simulink model "test"  (R2023a)
settings: Solver=FixedStepAuto  StartTime=0.0  StopTime=1  FixedStep=1e-4  MaxStep=1e-4  MinStep=1e-5  RelTol=1e-6  AbsTol=1e-5
values from neighbouring files (symbols this model uses):
  abc_alpha_beta = sqrt(2/3) * [1, -1/2, -1/2 ... (first row only)    [main.m]
  Flux_1 = 1/(Msr^2 - Ls * Lr )  * [Rs*Lr, 0, -Rs*Msr, 0 ... (first row only)    [main.m]
  Flux_2 = 1/(Msr^2 - Ls * Lr )  * [0, 0, 0, 0 ... (first row only)    [main.m]
  frot = 0.01    [main.m]
  Inv_abc_alpha_beta = inv(abc_alpha_beta)    [main.m]
  Inv_Phi_Courant = inv(Phi_Courant)    [main.m]
  J = 0.025    [main.m]
  Lr = 0.194    [main.m]
  Ls = 0.182    [main.m]
  Msr = 0.182    [main.m]
  p = 2    [main.m]
  Rr = 1.15    [main.m]
  Rs = 1.6    [main.m]
  T_charge = 0    [main.m]
  Vn = 380    [main.m]
settings Model: Creator=philippecasteres  LastModifiedBy=philippecasteres

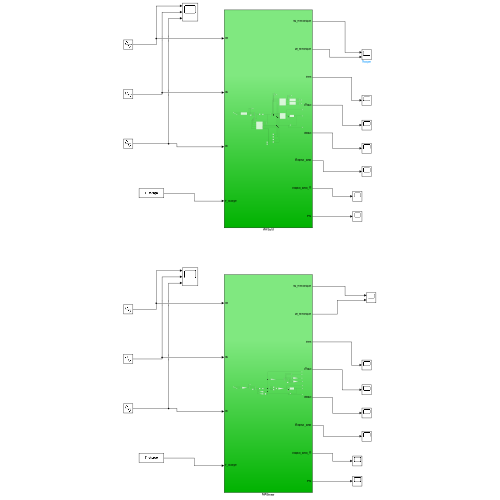
[thumbnail: Simulink's stored preview of the top-level diagram]
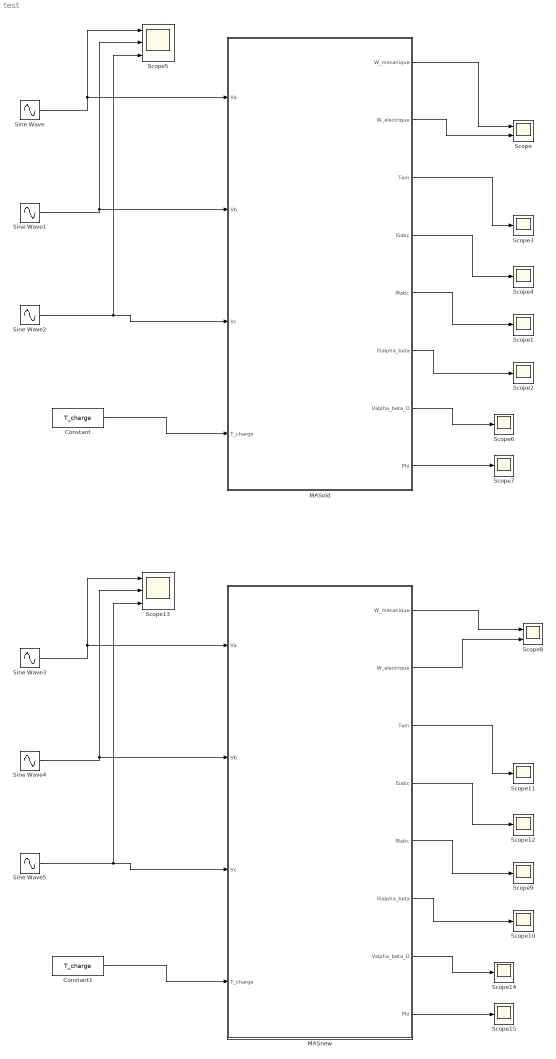
== system test ==
  Constant : Constant  Value=T_charge
  Constant1 : Constant  Value=T_charge
  MASnew : Subsystem
  MASold : Subsystem
  Scope : Scope  NumInputPorts=2
  Scope{1..4,6..7,9..12,14..15} (12 alike) : Scope
  Scope13 : Scope  NumInputPorts=3
  Scope5 : Scope  NumInputPorts=3
  Scope8 : Scope  NumInputPorts=2
  Sine Wave : Sin  Amplitude=Vn  Frequency=50*2*pi  SampleTime=0
  Sine Wave1 : Sin  Amplitude=Vn  Frequency=50*2*pi  Phase=-2*pi/3  SampleTime=0
  Sine Wave2 : Sin  Amplitude=Vn  Frequency=50*2*pi  Phase=-4*pi/3  SampleTime=0
  Sine Wave3 : Sin  Amplitude=Vn  Frequency=50*2*pi  SampleTime=0
  Sine Wave4 : Sin  Amplitude=Vn  Frequency=50*2*pi  Phase=-2*pi/3  SampleTime=0
  Sine Wave5 : Sin  Amplitude=Vn  Frequency=50*2*pi  Phase=-4*pi/3  SampleTime=0
  wires:
  Sine Wave2/1 -> Scope5/3, MASold/3(Vc)
  Sine Wave1/1 -> Scope5/2, MASold/2(Vb)
  Sine Wave/1 -> Scope5/1, MASold/1(Va)
  MASold/1(W_mecanique) -> Scope/1
  MASold/2(W_electrique) -> Scope/2
  MASold/3(Tem) -> Scope3/1
  Constant/1 -> MASold/4(T_charge)
  MASold/4(ISabc) -> Scope4/1
  MASold/5(IRabc) -> Scope1/1
  MASold/6(ISalpha_beta) -> Scope2/1
  MASold/7(Valpha_beta_O) -> Scope6/1
  MASold/8(Phi) -> Scope7/1
  MASnew/2(W_electrique) -> Scope8/2
  Sine Wave3/1 -> MASnew/1(Va), Scope13/1
  MASnew/1(W_mecanique) -> Scope8/1
  Sine Wave4/1 -> MASnew/2(Vb), Scope13/2
  MASnew/3(Tem) -> Scope11/1
  Constant1/1 -> MASnew/4(T_charge)
  Sine Wave5/1 -> MASnew/3(Vc), Scope13/3
  MASnew/4(ISabc) -> Scope12/1
  MASnew/7(Valpha_beta_O) -> Scope14/1
  MASnew/5(IRabc) -> Scope9/1
  MASnew/6(ISalpha_beta) -> Scope10/1
  MASnew/8(Phi) -> Scope15/1

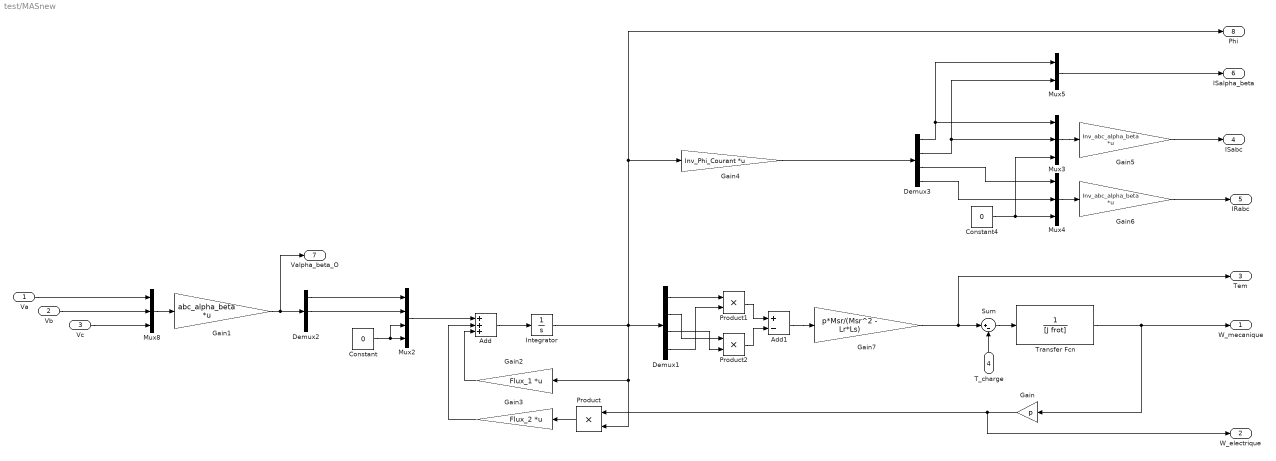
== system test/MASnew ==
  Va : Inport
  Vb : Inport  Port=2
  Vc : Inport  Port=3
  T_charge : Inport  Port=4
  Add : Sum  Inputs=+++
  Add1 : Sum  Inputs=+-
  Constant : Constant  Value=0
  Constant4 : Constant  Value=0
  Demux1 : Demux
  Demux2 : Demux  Outputs=3
  Demux3 : Demux
  Gain : Gain  Gain=p
  Gain1 : Gain  Gain=abc_alpha_beta  Multiplication=Matrix(K*u)
  Gain2 : Gain  Gain=Flux_1  Multiplication=Matrix(K*u)
  Gain3 : Gain  Gain=Flux_2  Multiplication=Matrix(K*u)
  Gain4 : Gain  Gain=Inv_Phi_Courant  Multiplication=Matrix(K*u)
  Gain5 : Gain  Gain=Inv_abc_alpha_beta  Multiplication=Matrix(K*u)
  Gain6 : Gain  Gain=Inv_abc_alpha_beta  Multiplication=Matrix(K*u)
  Gain7 : Gain  Gain=p*Msr/(Msr^2 - Lr*Ls)
  Integrator : Integrator
  Mux2 : Mux
  Mux3 : Mux  Inputs=3
  Mux4 : Mux  Inputs=3
  Mux5 : Mux  Inputs=2
  Mux8 : Mux  Inputs=3
  Product : Product
  Product1 : Product
  Product2 : Product
  Sum : Sum  Inputs=|+-
  Transfer Fcn : TransferFcn  Denominator=[J frot]
  W_mecanique : Outport
  W_electrique : Outport  Port=2
  Tem : Outport  Port=3
  ISabc : Outport  Port=4
  IRabc : Outport  Port=5
  ISalpha_beta : Outport  Port=6
  Valpha_beta_O : Outport  Port=7
  Phi : Outport  Port=8
  wires:
  Demux3/4 -> Mux4/2
  Demux3/2 -> Mux3/2, Mux5/2
  T_charge/1 -> Sum/2
  Demux3/1 -> Mux3/1, Mux5/1
  Va/1 -> Mux8/1
  Sum/1 -> Transfer Fcn/1
  Demux1/1 -> Product1/1
  Demux3/3 -> Mux4/1
  Gain7/1 -> Sum/1, Tem/1
  Transfer Fcn/1 -> Gain/1, W_mecanique/1
  Add/1 -> Integrator/1
  Vc/1 -> Mux8/3
  Vb/1 -> Mux8/2
  Product/1 -> Gain3/1
  Integrator/1 -> Gain2/1, Product/2, Demux1/1, Gain4/1, Phi/1
  Mux2/1 -> Add/1
  Mux3/1 -> Gain5/1
  Mux5/1 -> ISalpha_beta/1
  Gain1/1 -> Valpha_beta_O/1, Demux2/1
  Mux8/1 -> Gain1/1
  Demux2/1 -> Mux2/1
  Demux2/2 -> Mux2/2
  Constant/1 -> Mux2/4, Mux2/3
  Gain2/1 -> Add/3
  Gain4/1 -> Demux3/1
  Constant4/1 -> Mux4/3, Mux3/3
  Gain5/1 -> ISabc/1
  Mux4/1 -> Gain6/1
  Gain6/1 -> IRabc/1
  Product1/1 -> Add1/1
  Product2/1 -> Add1/2
  Add1/1 -> Gain7/1
  Gain/1 -> W_electrique/1, Product/1
  Gain3/1 -> Add/2
  Demux1/4 -> Product1/2
  Demux1/2 -> Product2/1
  Demux1/3 -> Product2/2

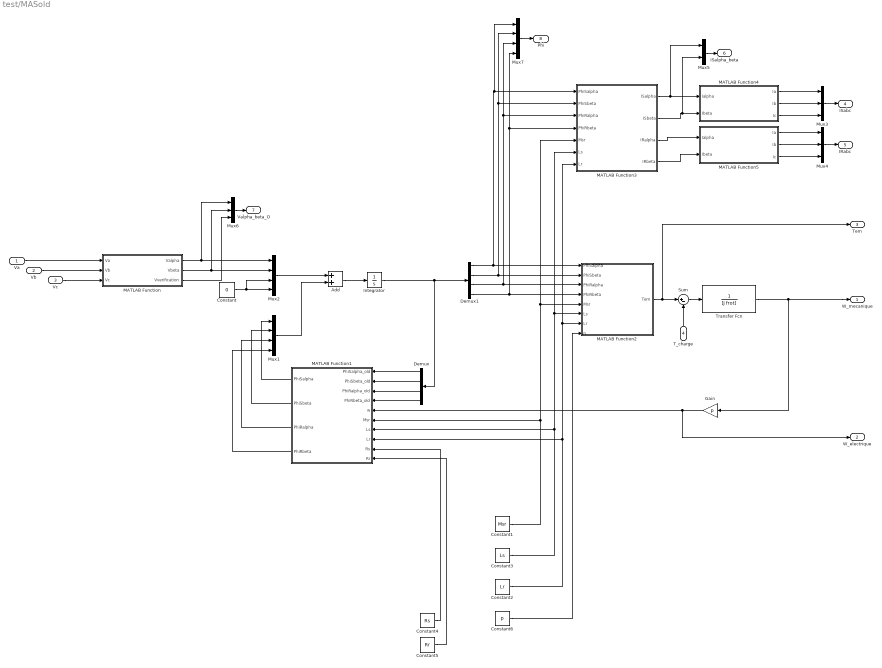
== system test/MASold ==
  Va : Inport
  Vb : Inport  Port=2
  Vc : Inport  Port=3
  T_charge : Inport  Port=4
  Add : Sum
  Constant : Constant  Value=0
  Constant1 : Constant  Value=Msr
  Constant2 : Constant  Value=Lr
  Constant3 : Constant  Value=Ls
  Constant4 : Constant  Value=Rs
  Constant5 : Constant  Value=Rr
  Constant6 : Constant  Value=p
  Demux : Demux
  Demux1 : Demux
  Gain : Gain  Gain=p
  Integrator : Integrator
  MATLAB Function : MATLAB Function  TreatAsAtomicUnit=on
  MATLAB Function1 : MATLAB Function  TreatAsAtomicUnit=on
  MATLAB Function2 : MATLAB Function  TreatAsAtomicUnit=on
  MATLAB Function3 : MATLAB Function  TreatAsAtomicUnit=on
  MATLAB Function4 : MATLAB Function  TreatAsAtomicUnit=on
  MATLAB Function5 : MATLAB Function  TreatAsAtomicUnit=on
  Mux1 : Mux
  Mux2 : Mux
  Mux3 : Mux  Inputs=3
  Mux4 : Mux  Inputs=3
  Mux5 : Mux  Inputs=2
  Mux6 : Mux  Inputs=3
  Mux7 : Mux
  Sum : Sum  Inputs=|+-
  Transfer Fcn : TransferFcn  Denominator=[J frot]
  W_mecanique : Outport
  W_electrique : Outport  Port=2
  Tem : Outport  Port=3
  ISabc : Outport  Port=4
  IRabc : Outport  Port=5
  ISalpha_beta : Outport  Port=6
  Valpha_beta_O : Outport  Port=7
  Phi : Outport  Port=8
  wires:
  MATLAB Function3/4(IRbeta) -> MATLAB Function5/2(Ibeta)
  MATLAB Function3/2(ISbeta) -> Mux5/2, MATLAB Function4/2(Ibeta)
  T_charge/1 -> Sum/2
  MATLAB Function3/1(ISalpha) -> Mux5/1, MATLAB Function4/1(Ialpha)
  Demux1/4 -> Mux7/4, MATLAB Function3/4(PhiRbeta), MATLAB Function2/4(PhiRbeta)
  Demux/2 -> MATLAB Function1/2(PhiSbeta_old)
  MATLAB Function1/3(PhiRalpha) -> Mux1/3
  Va/1 -> MATLAB Function/1(Va)
  Demux/3 -> MATLAB Function1/3(PhiRalpha_old)
  Sum/1 -> Transfer Fcn/1
  Demux1/1 -> Mux7/1, MATLAB Function3/1(PhiSalpha), MATLAB Function2/1(PhiSalpha)
  MATLAB Function1/1(PhiSalpha) -> Mux1/1
  Demux1/3 -> Mux7/3, MATLAB Function3/3(PhiRalpha), MATLAB Function2/3(PhiRalpha)
  MATLAB Function3/3(IRalpha) -> MATLAB Function5/1(Ialpha)
  MATLAB Function1/4(PhiRbeta) -> Mux1/4
  MATLAB Function2/1(Tem) -> Tem/1, Sum/1
  Transfer Fcn/1 -> W_mecanique/1, Gain/1
  Add/1 -> Integrator/1
  Gain/1 -> W_electrique/1, MATLAB Function1/5(w)
  Demux1/2 -> Mux7/2, MATLAB Function3/2(PhiSbeta), MATLAB Function2/2(PhiSbeta)
  Demux/4 -> MATLAB Function1/4(PhiRbeta_old)
  MATLAB Function1/2(PhiSbeta) -> Mux1/2
  Demux/1 -> MATLAB Function1/1(PhiSalpha_old)
  Vc/1 -> MATLAB Function/3(Vc)
  Vb/1 -> MATLAB Function/2(Vb)
  Mux1/1 -> Add/2
  Integrator/1 -> Demux1/1, Demux/1
  Constant/1 -> Mux2/4, Mux2/3
  Mux2/1 -> Add/1
  Constant1/1 -> MATLAB Function1/6(Msr), MATLAB Function3/5(Msr), MATLAB Function2/5(Msr)
  Constant3/1 -> MATLAB Function1/7(Ls), MATLAB Function3/6(Ls), MATLAB Function2/6(Ls)
  Constant2/1 -> MATLAB Function1/8(Lr), MATLAB Function3/7(Lr), MATLAB Function2/7(Lr)
  Constant4/1 -> MATLAB Function1/9(Rs)
  Constant5/1 -> MATLAB Function1/10(Rr)
  Constant6/1 -> MATLAB Function2/8(p)
  MATLAB Function5/1(Ia) -> Mux4/1
  MATLAB Function5/2(Ib) -> Mux4/2
  MATLAB Function5/3(Ic) -> Mux4/3
  MATLAB Function4/2(Ib) -> Mux3/2
  MATLAB Function4/1(Ia) -> Mux3/1
  MATLAB Function4/3(Ic) -> Mux3/3
  Mux3/1 -> ISabc/1
  Mux4/1 -> IRabc/1
  Mux5/1 -> ISalpha_beta/1
  MATLAB Function/2(Vbeta) -> Mux2/2, Mux6/2
  MATLAB Function/1(Valpha) -> Mux6/1, Mux2/1
  Mux6/1 -> Valpha_beta_O/1
  MATLAB Function/3(Vverification) -> Mux6/3
  Mux7/1 -> Phi/1

== matlab function test/MASold/MATLAB Function1 ==
  data: PhiSalpha_old input; PhiSalpha output; PhiSbeta_old input; PhiSbeta output; PhiRalpha output; PhiRbeta output; PhiRalpha_old input; PhiRbeta_old input; w input; Msr input; Ls input; Lr input; Rs input; Rr input
function [PhiSalpha,PhiSbeta,PhiRalpha,PhiRbeta] =Flux_Flux(PhiSalpha_old,PhiSbeta_old,PhiRalpha_old,PhiRbeta_old,w, Msr, Ls, Lr, Rs, Rr)

    PHI=[PhiSalpha_old;PhiSbeta_old;PhiRalpha_old;PhiRbeta_old];
    % Matrice de transformation
    transformation_matrix = 1/(Msr^2 - Ls * Lr )  * [Rs*Lr, 0, -Rs*Msr, 0;
                                                    0, Rs*Lr, 0, -Rs*Msr;
                                                    -Rr*Msr, 0, Rr*Ls, -w*(Msr^2 -Ls*Lr);
                                                    0, -Rr*Msr,w*(Msr^2 -Ls*Lr), Rr*Ls];
    
    % Calcul des résultats
    result = transformation_matrix * PHI;
    
    % Attribution des résultats aux sorties
    PhiSalpha = result(1);
    PhiSbeta = result(2);
    PhiRalpha = result(3);
    PhiRbeta = result(4);
end

== matlab function test/MASold/MATLAB Function ==
  data: Va input; Valpha output; Vb input; Vc input; Vbeta output; Vverification output
function [Valpha, Vbeta, Vverification] = abc_alpha_beta(Va, Vb, Vc)
    % Entrée : Va, Vb, Vc (les tensions de phase)
    % Sortie : Valpha, Vbeta, Vverification (les tensions transformées)
    
    % Vecteur de tensions d'entrée
    V = [Va; Vb; Vc];
    
    % Matrice de transformation
    transformation_matrix = sqrt(2/3) * [1 -1/2 -1/2;
                                          0 sqrt(3)/2 -sqrt(3)/2;
                                          1/sqrt(2) 1/sqrt(2) 1/sqrt(2)];
    
    % Calcul des résultats
    result = transformation_matrix * V;
    
    % Attribution des résultats aux sorties
    Valpha = result(1);
    Vbeta = result(2);
    Vverification = result(3);
end

== matlab function test/MASold/MATLAB Function2 ==
  data: PhiSalpha input; Tem output; PhiSbeta input; PhiRalpha input; PhiRbeta input; Msr input; Ls input; Lr input; p input
function Tem = Couple_em(PhiSalpha,PhiSbeta,PhiRalpha,PhiRbeta, Msr, Ls, Lr,p)

Tem = p*Msr/(Msr^2 - Lr*Ls)*(PhiSalpha * PhiRbeta - PhiRalpha * PhiSbeta);
end

== matlab function test/MASold/MATLAB Function3 ==
  data: PhiSalpha input; ISalpha output; PhiSbeta input; PhiRalpha input; PhiRbeta input; ISbeta output; IRalpha output; IRbeta output; Msr input; Ls input; Lr input
function [ISalpha, ISbeta, IRalpha, IRbeta] = Phi_Courant(PhiSalpha, PhiSbeta, PhiRalpha, PhiRbeta, Msr, Ls, Lr)
    % Entrée : 
    % PhiSalpha, PhiSbeta, PhiRalpha, PhiRbeta (flux)
    % Ls : inductance statorique
    % Lr : inductance rotorique
    % Msr : inductance mutuelle entre stator et rotor

    % Vecteur des flux d'entrée
    Phi = [PhiSalpha; PhiSbeta; PhiRalpha; PhiRbeta];

    % Matrice de transformation avec paramètres d'inductance
    transformation_matrix = [Ls,  0,   Msr,  0;
                             0,   Ls,  0,   Msr;
                             Msr, 0,   Lr,  0;
                             0,   Msr, 0,   Lr];

    % Calcul des résultats
    result = transformation_matrix \ Phi;  % Utilisation de la division matricielle pour inverser la matrice

    % Attribution des résultats aux sorties
    ISalpha = result(1);
    ISbeta = result(2);
    IRalpha = result(3);
    IRbeta = result(4);
end

== matlab function test/MASold/MATLAB Function4 ==
  data: Ialpha input; Ia output; Ibeta input; Ib output; Ic output
function [Ia, Ib, Ic] = alpha_beta_abc(Ialpha, Ibeta)

    % Vecteur de courants d'entrée (ajout de Io = 0 pour compléter le vecteur)
    I = [Ialpha; Ibeta; 0];
    
    % Matrice de transformation (de abc à alpha-beta)
    transformation_matrix = sqrt(2/3) * [1, -1/2, -1/2;
                                          0, sqrt(3)/2, -sqrt(3)/2;
                                          1/sqrt(2), 1/sqrt(2), 1/sqrt(2)];
    
    % Calcul des résultats via l'inversion de la matrice de transformation
    result = inv(transformation_matrix) * I;
    
    % Attribution des résultats aux sorties
    Ia = result(1);
    Ib = result(2);
    Ic = result(3);
end

== matlab function test/MASold/MATLAB Function5 ==
  data: Ialpha input; Ia output; Ibeta input; Ib output; Ic output
function [Ia, Ib, Ic] = alpha_beta_abc(Ialpha, Ibeta)

    % Vecteur de courants d'entrée (ajout de Io = 0 pour compléter le vecteur)
    I = [Ialpha; Ibeta; 0];
    
    % Matrice de transformation (de abc à alpha-beta)
    transformation_matrix = sqrt(2/3) * [1, -1/2, -1/2;
                                          0, sqrt(3)/2, -sqrt(3)/2;
                                          1/sqrt(2), 1/sqrt(2), 1/sqrt(2)];
    
    % Calcul des résultats via l'inversion de la matrice de transformation
    result = inv(transformation_matrix) * I;
    
    % Attribution des résultats aux sorties
    Ia = result(1);
    Ib = result(2);
    Ic = result(3);
end
